simulink model "SD_NL_TORA2"  (R2019b)
settings: Solver=ode4  StartTime=0.0  StopTime=stoptime  FixedStep=h  RelTol=1e-6  AbsTol=1e-6  EnableMultiTasking=on
values from neighbouring files (symbols this model uses):
  A = [0, 1, 0, 0 ... (first row only)    [mainfile_solution.m]
  B = [0 ... (first row only)    [mainfile_solution.m]
  C = eye(4)    [mainfile_solution.m]
  D = zeros(4,1)    [mainfile_solution.m]
  J = 0.0002175    [mainfile_solution.m]
  k = 186.3    [mainfile_solution.m]
  Kd = place(Ad,Bd,p_z)    [mainfile_solution.m]
  L = 1    [mainfile_solution.m]
  M = 1.3608    [mainfile_solution.m]
  m = 0.096    [mainfile_solution.m]
  x0 = [20*pi/180 , 0 ,  0.1 , 0]'    [mainfile_solution.m]
  x0_tilde = x0 - x_bar    [mainfile_solution.m]
  x_bar = [0 0 0 0]'    [mainfile_solution.m]
settings Model: Creator=Ale  LastModifiedBy=don
settings SolverCC: AutoScaleAbsTol=off
settings DataIOCC: SaveFormat=Array  SignalLoggingSaveFormat=ModelDataLogs  SaveOutput=off  SaveTime=off  TimeSaveName=t
settings OptimizationCC: ExpressionDepthLimit=2147483647  LifeSpan=inf
settings DebuggingCC: UnderspecifiedInitializationDetection=Classic  MergeDetectMultiDrivingBlocksExec=none  FcnCallInpInsideContextMsg=warning  StateNameClashWarn=warning  SFUnexpectedBacktrackingDiag=warning  SFNoUnconditionalDefaultTransitionDiag=warning  SFExecutionAtInitializationDiag=none  ArithmeticOperatorsInVariantConditions=warning
settings HardwareCC: ProdBitPerPointer=32  ProdBitPerSizeT=32  ProdBitPerPtrDiffT=32  ProdLargestAtomicFloat=None  ProdIntDivRoundTo=Undefined  ProdEndianess=Unspecified  ProdWordSize=32  ProdHWDeviceType=32-bit Generic
settings ModelReferenceCC: PropagateSignalLabelsOutOfModel=off
settings SFSimCC: SimUseLocalCustomCode=off  CustomCodeUndefinedFunction=UseInterfaceOnly
settings RTWCC: RTWUseLocalCustomCode=off
settings CodeAppCC: StateflowObjectComments=on
settings GRTTargetCC: TargetLangStandard=C89/C90 (ANSI)  GeneratePreprocessorConditionals=Disable all  CombineOutputUpdateFcns=off  GRTInterface=on
settings ConfigComp: CovMetricSettings=dw  CovHtmlReporting=on  CovSaveCumulativeToWorkspaceVar=on  CovSaveSingleToWorkspaceVar=on  CovExternalEMLEnable=off

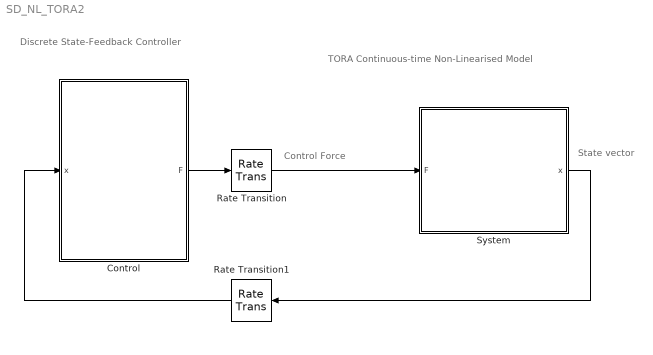
== system SD_NL_TORA2 ==
  note: Discrete State-Feedback
      | Controller
  note: Control Force
  note: State vector
  note: TORA
      | Continuous-time Non-Linearised Model
  Control : Subsystem
  Rate Transition : RateTransition  InitialCondition=-Kd*x0_tilde
  Rate Transition1 : RateTransition  InitialCondition=x0_tilde  OutPortSampleTime=Ts
  System : Subsystem
  wires:
  Control/1(F) -> Rate Transition/1
  Rate Transition/1 -> System/1(F)
  System/1(x) -> Rate Transition1/1
  Rate Transition1/1 -> Control/1(x)

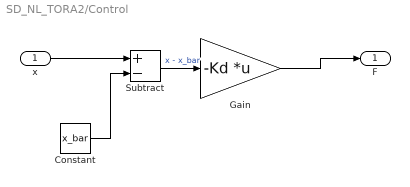
== system SD_NL_TORA2/Control ==
  x : Inport
  Constant : Constant  Value=x_bar
  Gain : Gain  Gain=-Kd  Multiplication=Matrix(K*u)
  Subtract : Sum  Inputs=+-
  F : Outport  VectorParamsAs1DForOutWhenUnconnected=off
  wires:
  Gain/1 -> F/1
  x/1 -> Subtract/1
  Constant/1 -> Subtract/2
  Subtract/1 -> Gain/1  "x - x_bar"

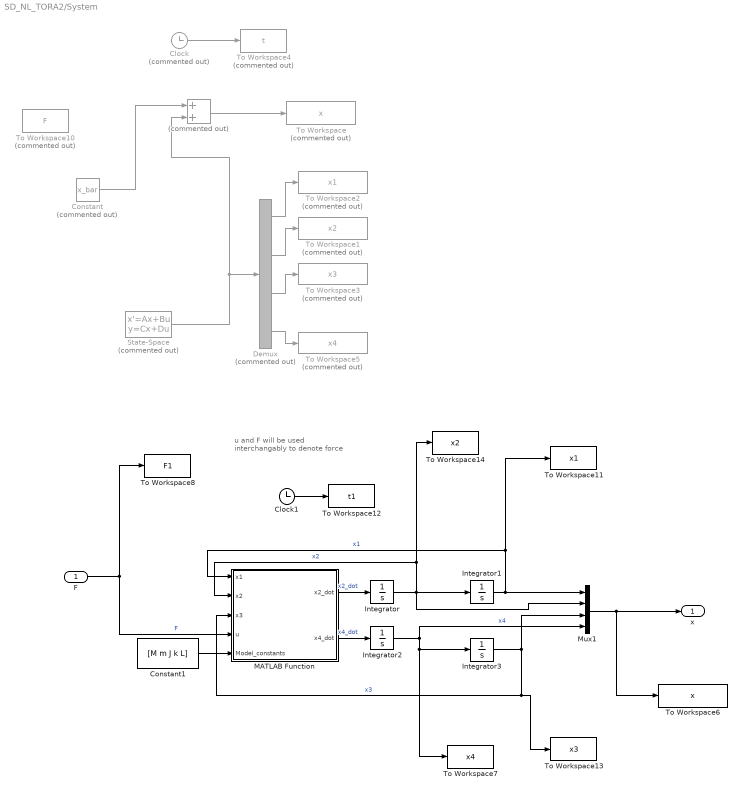
== system SD_NL_TORA2/System ==
  note: u and F will be used
      | interchangably to denote force
  F : Inport
  " " : Sum  Commented=on
  Clock : Clock  Commented=on
  Clock1 : Clock
  Constant : Constant  Commented=on  Value=x_bar
  Constant1 : Constant  Value=[M m J k L]
  Demux : Demux  Commented=on
  Integrator : Integrator  InitialCondition=x0(2)
  Integrator1 : Integrator  InitialCondition=x0(1)
  Integrator2 : Integrator  InitialCondition=x0(4)
  Integrator3 : Integrator  InitialCondition=x0(3)
  MATLAB Function : MATLAB Function  TreatAsAtomicUnit=on
  Mux1 : Mux
  State-Space : StateSpace  Commented=on  A=A  B=B  C=C  D=D  InitialCondition=x0
  To Workspace : ToWorkspace  Commented=on  VariableName=x  SampleTime=-1
  To Workspace1 : ToWorkspace  Commented=on  VariableName=x2  SampleTime=-1
  To Workspace10 : ToWorkspace  Commented=on  VariableName=F  SampleTime=-1
  To Workspace11 : ToWorkspace  VariableName=x1  SampleTime=-1
  To Workspace12 : ToWorkspace  VariableName=t1  SampleTime=-1
  To Workspace13 : ToWorkspace  VariableName=x3  SampleTime=-1
  To Workspace14 : ToWorkspace  VariableName=x2  SampleTime=-1
  To Workspace2 : ToWorkspace  Commented=on  VariableName=x1  SampleTime=-1
  To Workspace3 : ToWorkspace  Commented=on  VariableName=x3  SampleTime=-1
  To Workspace4 : ToWorkspace  Commented=on  VariableName=t  SampleTime=-1
  To Workspace5 : ToWorkspace  Commented=on  VariableName=x4  SampleTime=-1
  To Workspace6 : ToWorkspace  VariableName=x  SampleTime=-1
  To Workspace7 : ToWorkspace  VariableName=x4  SampleTime=-1
  To Workspace8 : ToWorkspace  VariableName=F1  SampleTime=-1
  x : Outport  VectorParamsAs1DForOutWhenUnconnected=off
  wires:
  State-Space/1 -> " "/2, Demux/1
  Clock/1 -> To Workspace4/1
  Constant/1 -> " "/1
  " "/1 -> To Workspace/1
  Demux/3 -> To Workspace3/1
  Demux/2 -> To Workspace1/1
  Demux/1 -> To Workspace2/1
  Demux/4 -> To Workspace5/1
  MATLAB Function/2(x4_dot) -> Integrator2/1  "x4_dot"
  Integrator3/1 -> To Workspace13/1, MATLAB Function/3(x3), Mux1/3  "x3"
  MATLAB Function/1(x2_dot) -> Integrator/1  "x2_dot"
  Integrator/1 -> Mux1/2, To Workspace14/1, MATLAB Function/2(x2), Integrator1/1  "x2"
  Integrator1/1 -> To Workspace11/1, MATLAB Function/1(x1), Mux1/1  "x1"
  Clock1/1 -> To Workspace12/1
  Constant1/1 -> MATLAB Function/5(Model_constants)
  Integrator2/1 -> Mux1/4, To Workspace7/1, Integrator3/1  "x4"
  Mux1/1 -> x/1, To Workspace6/1
  F/1 -> MATLAB Function/4(u), To Workspace8/1  "F"

== matlab function SD_NL_TORA2/System/MATLAB Function ==
  data: x1 input; x2_dot output; x2 input; x3 input; u input; x4_dot output; Model_constants input
function [x2_dot,x4_dot] = NonLinearEquations(x1,x2,x3,u,Model_constants)

%Get Model Constants:
M = Model_constants(1);
m = Model_constants(2);
J = Model_constants(3);
k = Model_constants(4);
L = Model_constants(5);

% Equation for x2_dot
x2_dot_nancy = (((m+M)*u)-(m*L*cos(x1)*(m*L*(x2^2)*sin(x1)-(k*(x3)))));
x2_dot_donkey = ((J+(m*(L^2))*(m+M))-((m^2)*(L^2)*cos(x1)^2));
x2_dot = x2_dot_nancy / x2_dot_donkey ;

% Equation for x2_dot
x4_dot_nancy = ((-m*L*u*cos(x1))+(J+(m*(L^2)))*(m*L*(x2^2)*sin(x1)-k*(x3)));
x4_dot_donkey = ((J+(m*(L^2))*(m+M))-((m^2)*L^2*cos(x1)^2));
x4_dot = x4_dot_nancy / x4_dot_donkey;

end
